simulink library "xrbsComm_r4"  (Simulink 7.1)
PreLoadFcn:
  | warning('off','MATLAB:mex:deprecatedExtension');xlmeta;com.xilinx.sysgen.util.StrategyUtil.loadAllStrategyNames();
undefined symbols (not defined in the file or in its folder): calc_path_data, gcbh, mfcm_matrix_rom, oct2dec, xlBlockLoadCallback
libraries: xbsIndex_r4 x851, mfcm_block_lib_v1 x5, xrbsComm_r4 x1, mfcm_misc_lib_v1 x1
(part 2 of 8)

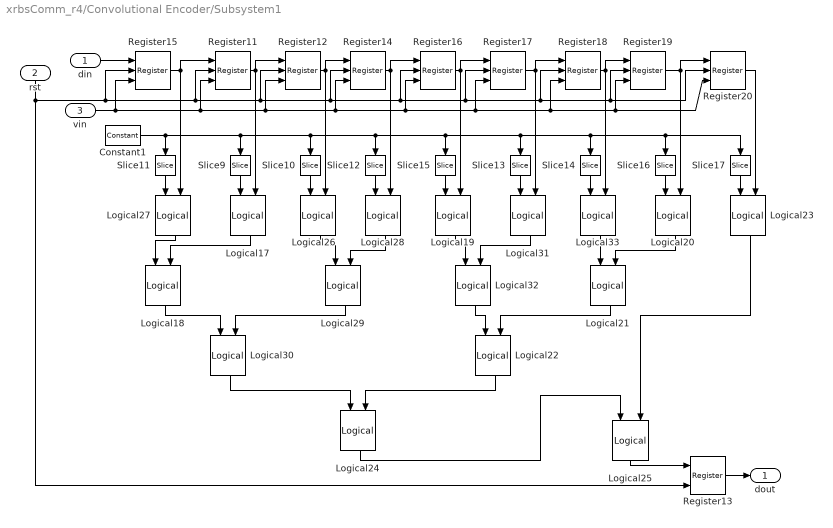
== system xrbsComm_r4/Convolutional Encoder/Subsystem1 ==
  din : Inport  OutDataType=sfix(16)  OutScaling=2^0
  rst : Inport  Orientation=down  Port=2  OutDataType=sfix(16)  OutScaling=2^0
  vin : Inport  Port=3  OutDataType=sfix(16)  OutScaling=2^0
  Constant1 : xbsIndex_r4/Constant  arith_type=Unsigned  const=oct2dec(code(index))*2^(9-K)  n_bits=9  bin_pt=0  explicit_period=off  period=1  equ=P=C  opselect=C  inp2=PCIN>>17  opr=+  inp1=P  carry=CIN  dbl_ovrd=off  block_type=constant
      settings: block_version=VER_STRING_GOES_HERE
  Logical{17,19..20,23,26..28,31,33} (9 alike) : xbsIndex_r4/Logical  Orientation=down  logical_function=AND  inputs=2  en=off  latency=0  precision=Full  arith_type=Unsigned  n_bits=16  bin_pt=0  align_bp=on  dbl_ovrd=off  block_type=logical
      settings: block_version=VER_STRING_GOES_HERE
  Logical{18,21..22,24..25,29..30,32} (8 alike) : xbsIndex_r4/Logical  Orientation=down  logical_function=XOR  inputs=2  en=off  latency=0  precision=Full  arith_type=Unsigned  n_bits=16  bin_pt=0  align_bp=on  dbl_ovrd=off  block_type=logical
      settings: block_version=VER_STRING_GOES_HERE
  Register{11..12,14..20} (9 alike) : xbsIndex_r4/Register  init=0  rst=on  en=on  dbl_ovrd=off  block_type=register
      settings: block_version=VER_STRING_GOES_HERE
  Register13 : xbsIndex_r4/Register  init=0  rst=on  en=off  dbl_ovrd=off  block_type=register
      settings: block_version=VER_STRING_GOES_HERE
  Slice10 : xbsIndex_r4/Slice  Orientation=down  nbits=1  boolean_output=off  mode=Upper Bit Location + Width  bit1=6  base1=LSB of Input  bit0=0  base0=LSB of Input  dbl_ovrd=off  block_type=slice
      settings: infoedit="Extracts a given range of bits from each input sample and presents it at the output.  The output type is ordinarily unsigned with binary point at zero, but can be Boolean when the slice is one bit wide.<P><P>Hardware notes: In hardware this block costs nothing."  block_version=VER_STRING_GOES_HERE
  Slice11 : xbsIndex_r4/Slice  Orientation=down  nbits=1  boolean_output=off  mode=Upper Bit Location + Width  bit1=8  base1=LSB of Input  bit0=0  base0=LSB of Input  dbl_ovrd=off  block_type=slice
      settings: infoedit="Extracts a given range of bits from each input sample and presents it at the output.  The output type is ordinarily unsigned with binary point at zero, but can be Boolean when the slice is one bit wide.<P><P>Hardware notes: In hardware this block costs nothing."  block_version=VER_STRING_GOES_HERE
  Slice12 : xbsIndex_r4/Slice  Orientation=down  nbits=1  boolean_output=off  mode=Upper Bit Location + Width  bit1=5  base1=LSB of Input  bit0=0  base0=LSB of Input  dbl_ovrd=off  block_type=slice
      settings: infoedit="Extracts a given range of bits from each input sample and presents it at the output.  The output type is ordinarily unsigned with binary point at zero, but can be Boolean when the slice is one bit wide.<P><P>Hardware notes: In hardware this block costs nothing."  block_version=VER_STRING_GOES_HERE
  Slice13 : xbsIndex_r4/Slice  Orientation=down  nbits=1  boolean_output=off  mode=Upper Bit Location + Width  bit1=3  base1=LSB of Input  bit0=0  base0=LSB of Input  dbl_ovrd=off  block_type=slice
      settings: infoedit="Extracts a given range of bits from each input sample and presents it at the output.  The output type is ordinarily unsigned with binary point at zero, but can be Boolean when the slice is one bit wide.<P><P>Hardware notes: In hardware this block costs nothing."  block_version=VER_STRING_GOES_HERE
  Slice14 : xbsIndex_r4/Slice  Orientation=down  nbits=1  boolean_output=off  mode=Upper Bit Location + Width  bit1=2  base1=LSB of Input  bit0=0  base0=LSB of Input  dbl_ovrd=off  block_type=slice
      settings: infoedit="Extracts a given range of bits from each input sample and presents it at the output.  The output type is ordinarily unsigned with binary point at zero, but can be Boolean when the slice is one bit wide.<P><P>Hardware notes: In hardware this block costs nothing."  block_version=VER_STRING_GOES_HERE
  Slice15 : xbsIndex_r4/Slice  Orientation=down  nbits=1  boolean_output=off  mode=Upper Bit Location + Width  bit1=4  base1=LSB of Input  bit0=0  base0=LSB of Input  dbl_ovrd=off  block_type=slice
      settings: infoedit="Extracts a given range of bits from each input sample and presents it at the output.  The output type is ordinarily unsigned with binary point at zero, but can be Boolean when the slice is one bit wide.<P><P>Hardware notes: In hardware this block costs nothing."  block_version=VER_STRING_GOES_HERE
  Slice16 : xbsIndex_r4/Slice  Orientation=down  nbits=1  boolean_output=off  mode=Upper Bit Location + Width  bit1=1  base1=LSB of Input  bit0=0  base0=LSB of Input  dbl_ovrd=off  block_type=slice
      settings: infoedit="Extracts a given range of bits from each input sample and presents it at the output.  The output type is ordinarily unsigned with binary point at zero, but can be Boolean when the slice is one bit wide.<P><P>Hardware notes: In hardware this block costs nothing."  block_version=VER_STRING_GOES_HERE
  Slice17 : xbsIndex_r4/Slice  Orientation=down  nbits=1  boolean_output=off  mode=Upper Bit Location + Width  bit1=0  base1=LSB of Input  bit0=0  base0=LSB of Input  dbl_ovrd=off  block_type=slice
      settings: infoedit="Extracts a given range of bits from each input sample and presents it at the output.  The output type is ordinarily unsigned with binary point at zero, but can be Boolean when the slice is one bit wide.<P><P>Hardware notes: In hardware this block costs nothing."  block_version=VER_STRING_GOES_HERE
  Slice9 : xbsIndex_r4/Slice  Orientation=down  nbits=1  boolean_output=off  mode=Upper Bit Location + Width  bit1=7  base1=LSB of Input  bit0=0  base0=LSB of Input  dbl_ovrd=off  block_type=slice
      settings: infoedit="Extracts a given range of bits from each input sample and presents it at the output.  The output type is ordinarily unsigned with binary point at zero, but can be Boolean when the slice is one bit wide.<P><P>Hardware notes: In hardware this block costs nothing."  block_version=VER_STRING_GOES_HERE
  dout : Outport  OutDataType=sfix(16)  OutScaling=2^0
  wires:
  Register12/1 -> Logical26/2, Register14/1
  Slice9/1 -> Logical17/1
  Slice10/1 -> Logical26/1
  Constant1/1 -> Slice9/1, Slice10/1, Slice12/1, Slice13/1, Slice14/1, Slice16/1, Slice17/1, Slice15/1, Slice11/1
  Slice11/1 -> Logical27/1
  Logical27/1 -> Logical18/1
  Logical17/1 -> Logical18/2
  Slice12/1 -> Logical28/1
  Logical26/1 -> Logical29/1
  Logical28/1 -> Logical29/2
  Logical18/1 -> Logical30/1
  Logical29/1 -> Logical30/2
  Register17/1 -> Logical31/2, Register18/1
  Register19/1 -> Logical20/2, Register20/1
  Register18/1 -> Register19/1, Logical33/2
  Slice13/1 -> Logical31/1
  Slice14/1 -> Logical33/1
  Slice15/1 -> Logical19/1
  Logical19/1 -> Logical32/1
  Logical31/1 -> Logical32/2
  Slice16/1 -> Logical20/1
  Logical33/1 -> Logical21/1
  Logical20/1 -> Logical21/2
  Logical32/1 -> Logical22/1
  Logical21/1 -> Logical22/2
  Register16/1 -> Logical19/2, Register17/1
  Register20/1 -> Logical23/2
  Slice17/1 -> Logical23/1
  Logical30/1 -> Logical24/1
  Logical22/1 -> Logical24/2
  Logical23/1 -> Logical25/2
  Logical24/1 -> Logical25/1
  Register15/1 -> Register11/1, Logical27/2
  Register14/1 -> Logical28/2, Register16/1
  Register11/1 -> Logical17/2, Register12/1
  Logical25/1 -> Register13/1
  din/1 -> Register15/1
  rst/1 -> Register11/2, Register16/2, Register18/2, Register20/2, Register19/2, Register17/2, Register14/2, Register12/2, Register15/2, Register13/2
  vin/1 -> Register20/3, Register19/3, Register18/3, Register17/3, Register16/3, Register14/3, Register12/3, Register11/3, Register15/3
  Register13/1 -> dout/1

== system xrbsComm_r4/Convolutional Encoder/Valid Out Logic ==
  vin : Inport  OutDataType=sfix(16)  OutScaling=2^0
  rst : Inport  Port=2  OutDataType=sfix(16)  OutScaling=2^0
  Register8 : xbsIndex_r4/Register  init=0  rst=on  en=off  dbl_ovrd=off  block_type=register
      settings: block_version=VER_STRING_GOES_HERE
  Register9 : xbsIndex_r4/Register  init=0  rst=on  en=off  dbl_ovrd=off  block_type=register
      settings: block_version=VER_STRING_GOES_HERE
  vout : Outport  OutDataType=sfix(16)  OutScaling=2^0
  wires:
  Register9/1 -> vout/1
  rst/1 -> Register9/2, Register8/2
  vin/1 -> Register8/1
  Register8/1 -> Register9/1

== system xrbsComm_r4/Multipath Fading Channel Model/matrix ops ==
  in_fd : Inport  OutDataType=sfix(16)  OutScaling=2^0
  in_rd : Inport  Port=2  OutDataType=sfix(16)  OutScaling=2^0
  in_reim : Inport  Port=3  OutDataType=sfix(16)  OutScaling=2^0
  fading_matrix : mfcm_block_lib_v1/fading_matrix  RATE=RATE  DATAPATH_WIDTH=DATAPATH_WIDTH  OUT_BINPT=FADE_BINPT  SPEC_DATA=SPEC_DATA  SEED=SEED
  matrix ROM : mfcm_block_lib_v1/matrix ROM  MATS=MATS  DATAPATH_WIDTH=DATAPATH_WIDTH  MAT_BINPT=MAT_BINPT
  rx_matrix : mfcm_block_lib_v1/rx_matrix  MR=size(RR,1)  N=length(GAIN)  BYPASS=MATS.rr_unity  WIDTH=DATAPATH_WIDTH  BINPT=RX_BINPT
  tx_matrix : mfcm_block_lib_v1/tx_matrix  MT=size(RT,1)  N=length(GAIN)  BYPASS=MATS.rt_unity  WIDTH=DATAPATH_WIDTH  BINPT=TX_BINPT
  out_fd : Outport  OutDataType=sfix(16)  OutScaling=2^0
  out_rd : Outport  Port=2  OutDataType=sfix(16)  OutScaling=2^0
  out_reim : Outport  Port=3  OutDataType=sfix(16)  OutScaling=2^0
  wires:
  tx_matrix/1 -> fading_matrix/1
  tx_matrix/2 -> fading_matrix/2
  tx_matrix/3 -> fading_matrix/3
  fading_matrix/1 -> rx_matrix/1
  fading_matrix/2 -> rx_matrix/2
  fading_matrix/3 -> rx_matrix/3
  rx_matrix/4 -> matrix ROM/1
  tx_matrix/4 -> matrix ROM/2
  matrix ROM/1 -> rx_matrix/4
  matrix ROM/2 -> tx_matrix/4
  rx_matrix/1 -> out_fd/1
  in_fd/1 -> tx_matrix/1
  rx_matrix/2 -> out_rd/1
  in_rd/1 -> tx_matrix/2
  rx_matrix/3 -> out_reim/1
  in_reim/1 -> tx_matrix/3

== system xrbsComm_r4/White Gaussian  Noise Generator/Box-Muller1 ==
  " reset" : Inport  OutDataType=sfix(16)  OutScaling=2^0
  Convert : xbsIndex_r4/Convert  arith_type="Signed  (2's comp)"  n_bits=10  bin_pt=6  quantization="Round  (unbiased: +/- Inf)"  overflow=Wrap  latency=2  dbl_ovrd=off  pipeline=off  block_type=convert
      settings: infoedit=The input is presented at the output after quantization and overflow effects.<P><P>Hardware notes: Additional hardware is used when rounding or saturation is selected and output width is less than the input width.  xl_area=[0, 0, 0, 0, 0, 0, 0]  block_version=VER_STRING_GOES_HERE
  Mult : xbsIndex_r4/Mult  precision=Full  arith_type="Signed  (2's comp)"  n_bits=20  bin_pt=0  quantization="Round  (unbiased: +/- Inf)"  overflow=Wrap  en=off  latency=2  dbl_ovrd=off  use_behavioral_HDL=off  use_embedded=on  pipeline=on  use_rpm=off  placement_style=Rectangular shape  block_type=mult
      settings: infoedit=Multiplies two values.<P><P>Hardware notes: To use the internal pipeline stage of the dedicated multiplier you must select 'Pipeline to Greatest Extent Possible'.  xl_area=[0, 0, 0, 0, 0, 0, 0]  block_version=VER_STRING_GOES_HERE
  f : Subsystem  mask(f_rom){init1=f_init1, init2=f_init2, init3=f_init3, init4=f_init4, init5=f_init5}
      mask prompts: init1 "init1(17:1)"; init2 "init2(25:1)"; init3 "init3(29:1)"; init4 "init4(31:1)"; init5 "init5(41:1)"
  g : Subsystem  mask{init=g_init}
      mask prompts: init "g_init(47:1)"
  bm : Outport  OutDataType=sfix(16)  OutScaling=2^0
  wires:
  g/1(g(s')) -> Mult/2
  f/1(f(s')) -> Mult/1
  Mult/1 -> Convert/1
  Convert/1 -> bm/1
  " reset"/1 -> f/1("reset "), g/1(reset)

== system xrbsComm_r4/White Gaussian  Noise Generator/Box-Muller2 ==
  reset : Inport  OutDataType=sfix(16)  OutScaling=2^0
  Convert : xbsIndex_r4/Convert  arith_type="Signed  (2's comp)"  n_bits=10  bin_pt=6  quantization="Round  (unbiased: +/- Inf)"  overflow=Wrap  latency=2  dbl_ovrd=off  pipeline=off  block_type=convert
      settings: infoedit=The input is presented at the output after quantization and overflow effects.<P><P>Hardware notes: Additional hardware is used when rounding or saturation is selected and output width is less than the input width.  xl_area=[0, 0, 0, 0, 0, 0, 0]  block_version=VER_STRING_GOES_HERE
  Mult : xbsIndex_r4/Mult  precision=Full  arith_type="Signed  (2's comp)"  n_bits=20  bin_pt=0  quantization="Round  (unbiased: +/- Inf)"  overflow=Wrap  en=off  latency=2  dbl_ovrd=off  use_behavioral_HDL=off  use_embedded=on  pipeline=on  use_rpm=off  placement_style=Rectangular shape  block_type=mult
      settings: infoedit=Multiplies two values.<P><P>Hardware notes: To use the internal pipeline stage of the dedicated multiplier you must select 'Pipeline to Greatest Extent Possible'.  xl_area=[0, 0, 0, 0, 0, 0, 0]  block_version=VER_STRING_GOES_HERE
  fr1 : Subsystem  mask(f_rom){init1=f_init1, init2=f_init2, init3=f_init3, init4=f_init4, init5=f_init5}
      mask prompts: init1 "init1(17:1)"; init2 "init2(25:1)"; init3 "init3(29:1)"; init4 "init4(31:1)"; init5 "init5(41:1)"
  g2 : Subsystem  mask{init=g_init}
      mask prompts: init "g_init(47:1)"
  bm : Outport  OutDataType=sfix(16)  OutScaling=2^0
  wires:
  g2/1(g(s')) -> Mult/2
  Mult/1 -> Convert/1
  Convert/1 -> bm/1
  reset/1 -> fr1/1(reset), g2/1(reset)
  fr1/1(f(s')) -> Mult/1

== system xrbsComm_r4/White Gaussian  Noise Generator/Box-Muller3 ==
  reset : Inport  OutDataType=sfix(16)  OutScaling=2^0
  Convert : xbsIndex_r4/Convert  arith_type="Signed  (2's comp)"  n_bits=10  bin_pt=6  quantization="Round  (unbiased: +/- Inf)"  overflow=Wrap  latency=2  dbl_ovrd=off  pipeline=off  block_type=convert
      settings: infoedit=The input is presented at the output after quantization and overflow effects.<P><P>Hardware notes: Additional hardware is used when rounding or saturation is selected and output width is less than the input width.  xl_area=[0, 0, 0, 0, 0, 0, 0]  block_version=VER_STRING_GOES_HERE
  Mult : xbsIndex_r4/Mult  precision=Full  arith_type="Signed  (2's comp)"  n_bits=20  bin_pt=0  quantization="Round  (unbiased: +/- Inf)"  overflow=Wrap  en=off  latency=2  dbl_ovrd=off  use_behavioral_HDL=off  use_embedded=on  pipeline=on  use_rpm=off  placement_style=Rectangular shape  block_type=mult
      settings: infoedit=Multiplies two values.<P><P>Hardware notes: To use the internal pipeline stage of the dedicated multiplier you must select 'Pipeline to Greatest Extent Possible'.  xl_area=[0, 0, 0, 0, 0, 0, 0]  block_version=VER_STRING_GOES_HERE
  fr1 : Subsystem  mask(f_rom){init1=f_init1, init2=f_init2, init3=f_init3, init4=f_init4, init5=f_init5}
      mask prompts: init1 "init1(17:1)"; init2 "init2(25:1)"; init3 "init3(29:1)"; init4 "init4(31:1)"; init5 "init5(41:1)"
  g2 : Subsystem  mask{init=g_init}
      mask prompts: init "g_init(47:1)"
  bm : Outport  OutDataType=sfix(16)  OutScaling=2^0
  wires:
  g2/1(g(s')) -> Mult/2
  fr1/1(f(s')) -> Mult/1
  Mult/1 -> Convert/1
  Convert/1 -> bm/1
  reset/1 -> fr1/1(reset), g2/1(reset)

== system xrbsComm_r4/White Gaussian  Noise Generator/Box-Muller4 ==
  reset : Inport  OutDataType=sfix(16)  OutScaling=2^0
  Convert : xbsIndex_r4/Convert  arith_type="Signed  (2's comp)"  n_bits=10  bin_pt=6  quantization="Round  (unbiased: +/- Inf)"  overflow=Wrap  latency=2  dbl_ovrd=off  pipeline=off  block_type=convert
      settings: infoedit=The input is presented at the output after quantization and overflow effects.<P><P>Hardware notes: Additional hardware is used when rounding or saturation is selected and output width is less than the input width.  xl_area=[0, 0, 0, 0, 0, 0, 0]  block_version=VER_STRING_GOES_HERE
  Mult : xbsIndex_r4/Mult  precision=Full  arith_type="Signed  (2's comp)"  n_bits=20  bin_pt=0  quantization="Round  (unbiased: +/- Inf)"  overflow=Wrap  en=off  latency=2  dbl_ovrd=off  use_behavioral_HDL=off  use_embedded=on  pipeline=on  use_rpm=off  placement_style=Rectangular shape  block_type=mult
      settings: infoedit=Multiplies two values.<P><P>Hardware notes: To use the internal pipeline stage of the dedicated multiplier you must select 'Pipeline to Greatest Extent Possible'.  xl_area=[0, 0, 0, 0, 0, 0, 0]  block_version=VER_STRING_GOES_HERE
  fr1 : Subsystem  mask(f_rom){init1=f_init1, init2=f_init2, init3=f_init3, init4=f_init4, init5=f_init5}
      mask prompts: init1 "init1(17:1)"; init2 "init2(25:1)"; init3 "init3(29:1)"; init4 "init4(31:1)"; init5 "init5(41:1)"
  g2 : Subsystem  mask{init=g_init}
      mask prompts: init "g_init(47:1)"
  bm : Outport  OutDataType=sfix(16)  OutScaling=2^0
  wires:
  reset/1 -> g2/1(reset), fr1/1(reset)
  g2/1(g(s')) -> Mult/2
  fr1/1(f(s')) -> Mult/1
  Mult/1 -> Convert/1
  Convert/1 -> bm/1

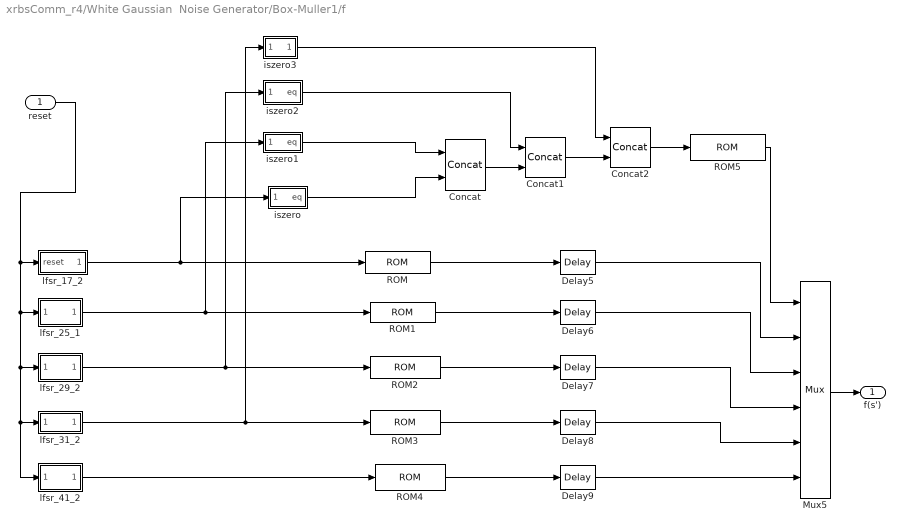
== system xrbsComm_r4/White Gaussian  Noise Generator/Box-Muller1/f ==
  "reset " : Inport  OutDataType=sfix(16)  OutScaling=2^0
  Concat : xbsIndex_r4/Concat  num_inputs=2  dbl_ovrd=off  block_type=concat
      settings: block_version=VER_STRING_GOES_HERE
  Concat1 : xbsIndex_r4/Concat  num_inputs=2  dbl_ovrd=off  block_type=concat
      settings: block_version=VER_STRING_GOES_HERE
  Concat2 : xbsIndex_r4/Concat  num_inputs=2  dbl_ovrd=off  block_type=concat
      settings: block_version=VER_STRING_GOES_HERE
  Delay{5..9} (5 alike) : xbsIndex_r4/Delay  en=off  latency=2  dbl_ovrd=off  reg_retiming=off  block_type=delay
      settings: infoedit="Delay line having  configurable length.<P><P>Hardware notes: A delay line is a chain, each link of which is an SRL16 followed by a flip-flop. If register retiming is enabled, the delay line is a chain of flip-flops."  xl_area=[0, 0, 0, 0, 0, 0, 0]  block_version=VER_STRING_GOES_HERE
  Mux5 : xbsIndex_r4/Mux  inputs=5  en=off  latency=1  precision=Full  arith_type="Signed  (2's comp)"  n_bits=10  bin_pt=0  quantization="Round  (unbiased: +/- Inf)"  overflow=Wrap  dbl_ovrd=off  block_type=mux
      settings: xl_area=[0, 0, 0, 0, 0, 0, 0]  block_version=VER_STRING_GOES_HERE
  ROM : xbsIndex_r4/ROM  depth=16  initVector=sqrt(-log( ((0:15)+0.51)'*(2.^(-1.*4)) ))  distributed_mem=Distributed memory  rst=off  init_reg=0  en=off  latency=1  arith_type=Unsigned  n_bits=9  bin_pt=7  dbl_ovrd=off  use_rpm=off  block_type=sprom
      settings: xl_area=[0, 0, 0, 0, 0, 0, 0]  block_version=VER_STRING_GOES_HERE
  ROM1 : xbsIndex_r4/ROM  depth=16  initVector=sqrt(-log( ((0:15)+0.51)'*(2.^(-2.*4)) ))  distributed_mem=Distributed memory  rst=off  init_reg=0  en=off  latency=1  arith_type=Unsigned  n_bits=9  bin_pt=7  dbl_ovrd=off  use_rpm=off  block_type=sprom
      settings: xl_area=[0, 0, 0, 0, 0, 0, 0]  block_version=VER_STRING_GOES_HERE
  ROM2 : xbsIndex_r4/ROM  depth=16  initVector=sqrt(-log( ((0:15)+0.51)'*(2.^(-3.*4)) ))  distributed_mem=Distributed memory  rst=off  init_reg=0  en=off  latency=1  arith_type=Unsigned  n_bits=9  bin_pt=7  dbl_ovrd=off  use_rpm=off  block_type=sprom
      settings: xl_area=[0, 0, 0, 0, 0, 0, 0]  block_version=VER_STRING_GOES_HERE
  ROM3 : xbsIndex_r4/ROM  depth=16  initVector=sqrt(-log( ((0:15)+0.51)'*(2.^(-4.*4)) ))  distributed_mem=Distributed memory  rst=off  init_reg=0  en=off  latency=1  arith_type=Unsigned  n_bits=9  bin_pt=7  dbl_ovrd=off  use_rpm=off  block_type=sprom
      settings: xl_area=[0, 0, 0, 0, 0, 0, 0]  block_version=VER_STRING_GOES_HERE
  ROM4 : xbsIndex_r4/ROM  depth=16  initVector=sqrt(-log( ((0:15)+0.51)'*(2.^(-5.*4)) ))  distributed_mem=Distributed memory  rst=off  init_reg=0  en=off  latency=1  arith_type=Unsigned  n_bits=9  bin_pt=7  dbl_ovrd=off  use_rpm=off  block_type=sprom
      settings: xl_area=[0, 0, 0, 0, 0, 0, 0]  block_version=VER_STRING_GOES_HERE
  ROM5 : xbsIndex_r4/ROM  depth=16  initVector=[0 1 0 2 0 1 0 3 0 1 0 2 0 1 0 4]  distributed_mem=Block RAM  rst=off  init_reg=0  en=off  latency=2  arith_type=Unsigned  n_bits=3  bin_pt=0  dbl_ovrd=off  use_rpm=off  block_type=sprom
      settings: xl_area=[0, 0, 0, 0, 0, 0, 0]  block_version=VER_STRING_GOES_HERE
  iszero : Subsystem
  iszero1 : Subsystem
  iszero2 : Subsystem
  iszero3 : Subsystem
  lfsr_17_2 : Subsystem  mask(lfsr_17){init=init1}
      mask prompts: init "init(17:1)"
  lfsr_25_1 : Subsystem  mask(lfsr_25){init=init2}
      mask prompts: init "init(25:1)"
  lfsr_29_2 : Subsystem  mask(lfsr_29){init=init3}
      mask prompts: init "init(29:1)"
  lfsr_31_2 : Subsystem  mask(lfsr_31){init=init4}
      mask prompts: init "init(31:1)"
  lfsr_41_2 : Subsystem  mask(lfsr_41){init=init5}
      mask prompts: init "init(41:1)"
  f(s') : Outport  OutDataType=sfix(16)  OutScaling=2^0
  wires:
  lfsr_17_2/1(" ") -> ROM/1, iszero/1(" ")
  lfsr_25_1/1(" ") -> ROM1/1, iszero1/1(" ")
  lfsr_29_2/1(" ") -> ROM2/1, iszero2/1(" ")
  lfsr_31_2/1(" ") -> iszero3/1(" "), ROM3/1
  lfsr_41_2/1(" ") -> ROM4/1
  Concat2/1 -> ROM5/1
  ROM5/1 -> Mux5/1
  Concat/1 -> Concat1/2
  Concat1/1 -> Concat2/2
  Mux5/1 -> f(s')/1
  ROM/1 -> Delay5/1
  ROM1/1 -> Delay6/1
  ROM2/1 -> Delay7/1
  ROM3/1 -> Delay8/1
  ROM4/1 -> Delay9/1
  iszero/1(eq) -> Concat/2
  iszero1/1(eq) -> Concat/1
  iszero2/1(eq) -> Concat1/1
  iszero3/1(eq) -> Concat2/1
  Delay5/1 -> Mux5/2
  Delay6/1 -> Mux5/3
  Delay7/1 -> Mux5/4
  Delay8/1 -> Mux5/5
  Delay9/1 -> Mux5/6
  "reset "/1 -> lfsr_25_1/1(" reset"), lfsr_41_2/1(reset), lfsr_31_2/1(reset), lfsr_29_2/1(reset), lfsr_17_2/1(reset)

== system xrbsComm_r4/White Gaussian  Noise Generator/Box-Muller1/g ==
  reset : Inport  OutDataType=sfix(16)  OutScaling=2^0
  Delay : xbsIndex_r4/Delay  en=off  latency=3  dbl_ovrd=off  reg_retiming=off  block_type=delay
      settings: infoedit="Delay line having  configurable length.<P><P>Hardware notes: A delay line is a chain, each link of which is an SRL16 followed by a flip-flop. If register retiming is enabled, the delay line is a chain of flip-flops."  xl_area=[0, 0, 0, 0, 0, 0, 0]  block_version=VER_STRING_GOES_HERE
  ROM : xbsIndex_r4/ROM  depth=256  initVector=sqrt(2) * cos(pi*((0:255) + 0.5)*2^(-8))  distributed_mem=Block RAM  rst=off  init_reg=0  en=off  latency=1  arith_type="Signed  (2's comp)"  n_bits=10  bin_pt=8  dbl_ovrd=off  use_rpm=off  block_type=sprom
      settings: xl_area=[0, 0, 0, 0, 0, 0, 0]  block_version=VER_STRING_GOES_HERE
  lfsr_47_5 : Subsystem  mask(lfsr_47){init=init}
      mask prompts: init "init(47:1)"
  g(s') : Outport  OutDataType=sfix(16)  OutScaling=2^0
  wires:
  ROM/1 -> Delay/1
  lfsr_47_5/1(" ") -> ROM/1
  Delay/1 -> g(s')/1
  reset/1 -> lfsr_47_5/1(reset)

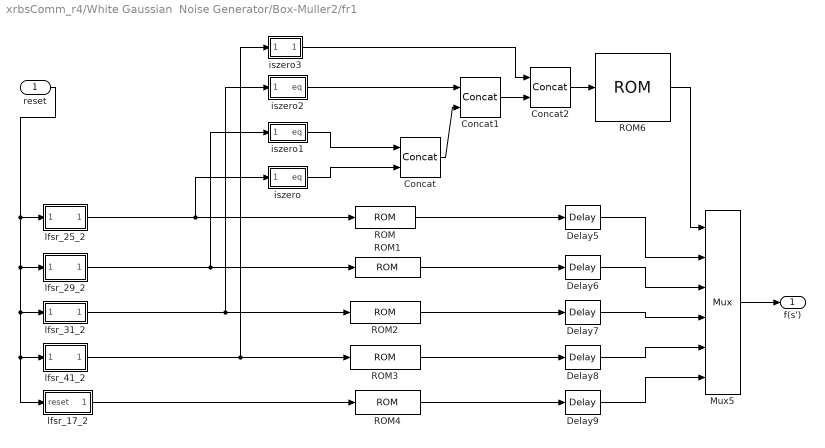
== system xrbsComm_r4/White Gaussian  Noise Generator/Box-Muller2/fr1 ==
  reset : Inport  OutDataType=sfix(16)  OutScaling=2^0
  Concat : xbsIndex_r4/Concat  num_inputs=2  dbl_ovrd=off  block_type=concat
      settings: block_version=VER_STRING_GOES_HERE
  Concat1 : xbsIndex_r4/Concat  num_inputs=2  dbl_ovrd=off  block_type=concat
      settings: block_version=VER_STRING_GOES_HERE
  Concat2 : xbsIndex_r4/Concat  num_inputs=2  dbl_ovrd=off  block_type=concat
      settings: block_version=VER_STRING_GOES_HERE
  Delay{5..9} (5 alike) : xbsIndex_r4/Delay  en=off  latency=2  dbl_ovrd=off  reg_retiming=off  block_type=delay
      settings: infoedit="Delay line having  configurable length.<P><P>Hardware notes: A delay line is a chain, each link of which is an SRL16 followed by a flip-flop. If register retiming is enabled, the delay line is a chain of flip-flops."  xl_area=[0, 0, 0, 0, 0, 0, 0]  block_version=VER_STRING_GOES_HERE
  Mux5 : xbsIndex_r4/Mux  inputs=5  en=off  latency=1  precision=Full  arith_type="Signed  (2's comp)"  n_bits=10  bin_pt=0  quantization="Round  (unbiased: +/- Inf)"  overflow=Wrap  dbl_ovrd=off  block_type=mux
      settings: xl_area=[0, 0, 0, 0, 0, 0, 0]  block_version=VER_STRING_GOES_HERE
  ROM : xbsIndex_r4/ROM  depth=16  initVector=sqrt(-log( ((0:15)+0.51)'*(2.^(-1.*4)) ))  distributed_mem=Distributed memory  rst=off  init_reg=0  en=off  latency=1  arith_type=Unsigned  n_bits=9  bin_pt=7  dbl_ovrd=off  use_rpm=off  block_type=sprom
      settings: xl_area=[0, 0, 0, 0, 0, 0, 0]  block_version=VER_STRING_GOES_HERE
  ROM1 : xbsIndex_r4/ROM  depth=16  initVector=sqrt(-log( ((0:15)+0.51)'*(2.^(-2.*4)) ))  distributed_mem=Distributed memory  rst=off  init_reg=0  en=off  latency=1  arith_type=Unsigned  n_bits=9  bin_pt=7  dbl_ovrd=off  use_rpm=off  block_type=sprom
      settings: xl_area=[0, 0, 0, 0, 0, 0, 0]  block_version=VER_STRING_GOES_HERE
  ROM2 : xbsIndex_r4/ROM  depth=16  initVector=sqrt(-log( ((0:15)+0.51)'*(2.^(-3.*4)) ))  distributed_mem=Distributed memory  rst=off  init_reg=0  en=off  latency=1  arith_type=Unsigned  n_bits=9  bin_pt=7  dbl_ovrd=off  use_rpm=off  block_type=sprom
      settings: xl_area=[0, 0, 0, 0, 0, 0, 0]  block_version=VER_STRING_GOES_HERE
  ROM3 : xbsIndex_r4/ROM  depth=16  initVector=sqrt(-log( ((0:15)+0.51)'*(2.^(-4.*4)) ))  distributed_mem=Distributed memory  rst=off  init_reg=0  en=off  latency=1  arith_type=Unsigned  n_bits=9  bin_pt=7  dbl_ovrd=off  use_rpm=off  block_type=sprom
      settings: xl_area=[0, 0, 0, 0, 0, 0, 0]  block_version=VER_STRING_GOES_HERE
  ROM4 : xbsIndex_r4/ROM  depth=16  initVector=sqrt(-log( ((0:15)+0.51)'*(2.^(-5.*4)) ))  distributed_mem=Distributed memory  rst=off  init_reg=0  en=off  latency=1  arith_type=Unsigned  n_bits=9  bin_pt=7  dbl_ovrd=off  use_rpm=off  block_type=sprom
      settings: xl_area=[0, 0, 0, 0, 0, 0, 0]  block_version=VER_STRING_GOES_HERE
  ROM6 : xbsIndex_r4/ROM  depth=16  initVector=[0 1 0 2 0 1 0 3 0 1 0 2 0 1 0 4]  distributed_mem=Block RAM  rst=off  init_reg=0  en=off  latency=2  arith_type=Unsigned  n_bits=3  bin_pt=0  dbl_ovrd=off  use_rpm=off  block_type=sprom
      settings: xl_area=[0, 0, 0, 0, 0, 0, 0]  block_version=VER_STRING_GOES_HERE
  iszero : Subsystem
  iszero1 : Subsystem
  iszero2 : Subsystem
  iszero3 : Subsystem
  lfsr_17_2 : Subsystem  mask(lfsr_17){init=init1}
      mask prompts: init "init(17:1)"
  lfsr_25_2 : Subsystem  mask(lfsr_25){init=init2}
      mask prompts: init "init(25:1)"
  lfsr_29_2 : Subsystem  mask(lfsr_29){init=init3}
      mask prompts: init "init(29:1)"
  lfsr_31_2 : Subsystem  mask(lfsr_31){init=init4}
      mask prompts: init "init(31:1)"
  lfsr_41_2 : Subsystem  mask(lfsr_41){init=init5}
      mask prompts: init "init(41:1)"
  f(s') : Outport  OutDataType=sfix(16)  OutScaling=2^0
  wires:
  Delay9/1 -> Mux5/6
  Delay8/1 -> Mux5/5
  Delay7/1 -> Mux5/4
  Delay6/1 -> Mux5/3
  Delay5/1 -> Mux5/2
  iszero/1(eq) -> Concat/2
  lfsr_25_2/1(" ") -> iszero/1(" "), ROM/1
  lfsr_29_2/1(" ") -> ROM1/1, iszero1/1(" ")
  lfsr_31_2/1(" ") -> iszero2/1(" "), ROM2/1
  lfsr_41_2/1(" ") -> ROM3/1, iszero3/1(" ")
  lfsr_17_2/1(" ") -> ROM4/1
  Concat/1 -> Concat1/2
  Concat1/1 -> Concat2/2
  ROM/1 -> Delay5/1
  ROM1/1 -> Delay6/1
  ROM4/1 -> Delay9/1
  ROM6/1 -> Mux5/1
  iszero1/1(eq) -> Concat/1
  Concat2/1 -> ROM6/1
  iszero2/1(eq) -> Concat1/1
  iszero3/1(eq) -> Concat2/1
  ROM2/1 -> Delay7/1
  ROM3/1 -> Delay8/1
  Mux5/1 -> f(s')/1
  reset/1 -> lfsr_25_2/1(" reset"), lfsr_29_2/1(reset), lfsr_31_2/1(reset), lfsr_17_2/1(reset), lfsr_41_2/1(reset)

== system xrbsComm_r4/White Gaussian  Noise Generator/Box-Muller2/g2 ==
  reset : Inport  OutDataType=sfix(16)  OutScaling=2^0
  Delay : xbsIndex_r4/Delay  en=off  latency=3  dbl_ovrd=off  reg_retiming=off  block_type=delay
      settings: infoedit="Delay line having  configurable length.<P><P>Hardware notes: A delay line is a chain, each link of which is an SRL16 followed by a flip-flop. If register retiming is enabled, the delay line is a chain of flip-flops."  xl_area=[0, 0, 0, 0, 0, 0, 0]  block_version=VER_STRING_GOES_HERE
  ROM : xbsIndex_r4/ROM  depth=256  initVector=sqrt(2) * cos(pi*((0:255) + 0.5)*2^(-8))  distributed_mem=Block RAM  rst=off  init_reg=0  en=off  latency=1  arith_type="Signed  (2's comp)"  n_bits=10  bin_pt=8  dbl_ovrd=off  use_rpm=off  block_type=sprom
      settings: xl_area=[0, 0, 0, 0, 0, 0, 0]  block_version=VER_STRING_GOES_HERE
  lfsr_47_5 : Subsystem  mask(lfsr_47){init=init}
      mask prompts: init "init(47:1)"
  g(s') : Outport  OutDataType=sfix(16)  OutScaling=2^0
  wires:
  ROM/1 -> Delay/1
  lfsr_47_5/1(" ") -> ROM/1
  Delay/1 -> g(s')/1
  reset/1 -> lfsr_47_5/1(reset)

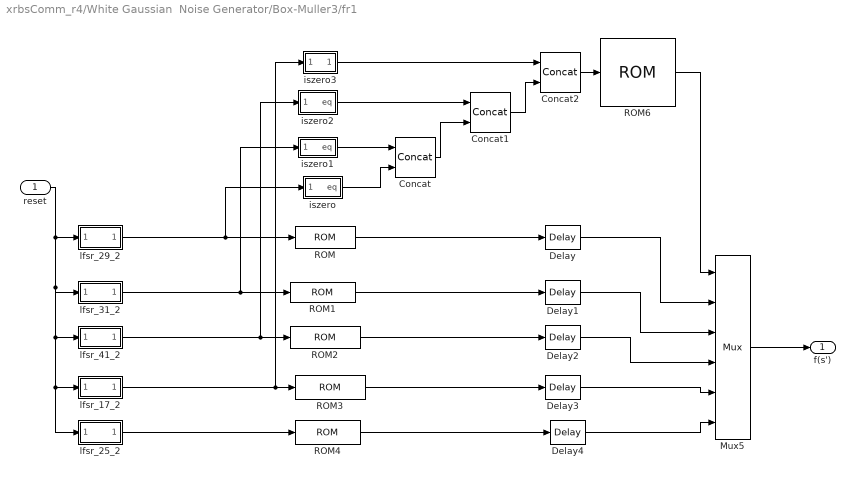
== system xrbsComm_r4/White Gaussian  Noise Generator/Box-Muller3/fr1 ==
  reset : Inport  OutDataType=sfix(16)  OutScaling=2^0
  Concat : xbsIndex_r4/Concat  num_inputs=2  dbl_ovrd=off  block_type=concat
      settings: block_version=VER_STRING_GOES_HERE
  Concat1 : xbsIndex_r4/Concat  num_inputs=2  dbl_ovrd=off  block_type=concat
      settings: block_version=VER_STRING_GOES_HERE
  Concat2 : xbsIndex_r4/Concat  num_inputs=2  dbl_ovrd=off  block_type=concat
      settings: block_version=VER_STRING_GOES_HERE
  Delay{,1..4} (5 alike) : xbsIndex_r4/Delay  en=off  latency=2  dbl_ovrd=off  reg_retiming=off  block_type=delay
      settings: infoedit="Delay line having  configurable length.<P><P>Hardware notes: A delay line is a chain, each link of which is an SRL16 followed by a flip-flop. If register retiming is enabled, the delay line is a chain of flip-flops."  xl_area=[0, 0, 0, 0, 0, 0, 0]  block_version=VER_STRING_GOES_HERE
  Mux5 : xbsIndex_r4/Mux  inputs=5  en=off  latency=1  precision=Full  arith_type="Signed  (2's comp)"  n_bits=10  bin_pt=0  quantization="Round  (unbiased: +/- Inf)"  overflow=Wrap  dbl_ovrd=off  block_type=mux
      settings: xl_area=[0, 0, 0, 0, 0, 0, 0]  block_version=VER_STRING_GOES_HERE
  ROM : xbsIndex_r4/ROM  depth=16  initVector=sqrt(-log( ((0:15)+0.51)'*(2.^(-1.*4)) ))  distributed_mem=Distributed memory  rst=off  init_reg=0  en=off  latency=1  arith_type=Unsigned  n_bits=9  bin_pt=7  dbl_ovrd=off  use_rpm=off  block_type=sprom
      settings: xl_area=[0, 0, 0, 0, 0, 0, 0]  block_version=VER_STRING_GOES_HERE
  ROM1 : xbsIndex_r4/ROM  depth=16  initVector=sqrt(-log( ((0:15)+0.51)'*(2.^(-2.*4)) ))  distributed_mem=Distributed memory  rst=off  init_reg=0  en=off  latency=1  arith_type=Unsigned  n_bits=9  bin_pt=7  dbl_ovrd=off  use_rpm=off  block_type=sprom
      settings: xl_area=[0, 0, 0, 0, 0, 0, 0]  block_version=VER_STRING_GOES_HERE
  ROM2 : xbsIndex_r4/ROM  depth=16  initVector=sqrt(-log( ((0:15)+0.51)'*(2.^(-3.*4)) ))  distributed_mem=Distributed memory  rst=off  init_reg=0  en=off  latency=1  arith_type=Unsigned  n_bits=9  bin_pt=7  dbl_ovrd=off  use_rpm=off  block_type=sprom
      settings: xl_area=[0, 0, 0, 0, 0, 0, 0]  block_version=VER_STRING_GOES_HERE
  ROM3 : xbsIndex_r4/ROM  depth=16  initVector=sqrt(-log( ((0:15)+0.51)'*(2.^(-4.*4)) ))  distributed_mem=Distributed memory  rst=off  init_reg=0  en=off  latency=1  arith_type=Unsigned  n_bits=9  bin_pt=7  dbl_ovrd=off  use_rpm=off  block_type=sprom
      settings: xl_area=[0, 0, 0, 0, 0, 0, 0]  block_version=VER_STRING_GOES_HERE
  ROM4 : xbsIndex_r4/ROM  depth=16  initVector=sqrt(-log( ((0:15)+0.51)'*(2.^(-5.*4)) ))  distributed_mem=Distributed memory  rst=off  init_reg=0  en=off  latency=1  arith_type=Unsigned  n_bits=9  bin_pt=7  dbl_ovrd=off  use_rpm=off  block_type=sprom
      settings: xl_area=[0, 0, 0, 0, 0, 0, 0]  block_version=VER_STRING_GOES_HERE
  ROM6 : xbsIndex_r4/ROM  depth=16  initVector=[0 1 0 2 0 1 0 3 0 1 0 2 0 1 0 4]  distributed_mem=Block RAM  rst=off  init_reg=0  en=off  latency=2  arith_type=Unsigned  n_bits=3  bin_pt=0  dbl_ovrd=off  use_rpm=off  block_type=sprom
      settings: xl_area=[0, 0, 0, 0, 0, 0, 0]  block_version=VER_STRING_GOES_HERE
  iszero : Subsystem
  iszero1 : Subsystem
  iszero2 : Subsystem
  iszero3 : Subsystem
  lfsr_17_2 : Subsystem  mask(lfsr_17){init=init1}
      mask prompts: init "init(17:1)"
  lfsr_25_2 : Subsystem  mask(lfsr_25){init=init2}
      mask prompts: init "init(25:1)"
  lfsr_29_2 : Subsystem  mask(lfsr_29){init=init3}
      mask prompts: init "init(29:1)"
  lfsr_31_2 : Subsystem  mask(lfsr_31){init=init4}
      mask prompts: init "init(31:1)"
  lfsr_41_2 : Subsystem  mask(lfsr_41){init=init5}
      mask prompts: init "init(41:1)"
  f(s') : Outport  OutDataType=sfix(16)  OutScaling=2^0
  wires:
  lfsr_29_2/1(" ") -> ROM/1, iszero/1(" ")
  lfsr_31_2/1(" ") -> ROM1/1, iszero1/1(" ")
  lfsr_41_2/1(" ") -> ROM2/1, iszero2/1(" ")
  lfsr_17_2/1(" ") -> iszero3/1(" "), ROM3/1
  lfsr_25_2/1(" ") -> ROM4/1
  Mux5/1 -> f(s')/1
  Concat/1 -> Concat1/2
  Concat1/1 -> Concat2/2
  Concat2/1 -> ROM6/1
  ROM6/1 -> Mux5/1
  ROM/1 -> Delay/1
  ROM1/1 -> Delay1/1
  ROM2/1 -> Delay2/1
  ROM3/1 -> Delay3/1
  ROM4/1 -> Delay4/1
  iszero/1(eq) -> Concat/2
  iszero1/1(eq) -> Concat/1
  iszero2/1(eq) -> Concat1/1
  iszero3/1(eq) -> Concat2/1
  Delay4/1 -> Mux5/6
  Delay3/1 -> Mux5/5
  Delay2/1 -> Mux5/4
  Delay1/1 -> Mux5/3
  Delay/1 -> Mux5/2
  reset/1 -> lfsr_31_2/1(reset), lfsr_41_2/1(reset), lfsr_25_2/1(" reset"), lfsr_17_2/1(reset), lfsr_29_2/1(reset)

== system xrbsComm_r4/White Gaussian  Noise Generator/Box-Muller3/g2 ==
  reset : Inport  OutDataType=sfix(16)  OutScaling=2^0
  Delay : xbsIndex_r4/Delay  en=off  latency=3  dbl_ovrd=off  reg_retiming=off  block_type=delay
      settings: infoedit="Delay line having  configurable length.<P><P>Hardware notes: A delay line is a chain, each link of which is an SRL16 followed by a flip-flop. If register retiming is enabled, the delay line is a chain of flip-flops."  xl_area=[0, 0, 0, 0, 0, 0, 0]  block_version=VER_STRING_GOES_HERE
  ROM : xbsIndex_r4/ROM  depth=256  initVector=sqrt(2) * cos(pi*((0:255) + 0.5)*2^(-8))  distributed_mem=Block RAM  rst=off  init_reg=0  en=off  latency=1  arith_type="Signed  (2's comp)"  n_bits=10  bin_pt=8  dbl_ovrd=off  use_rpm=off  block_type=sprom
      settings: xl_area=[0, 0, 0, 0, 0, 0, 0]  block_version=VER_STRING_GOES_HERE
  lfsr_47_5 : Subsystem  mask(lfsr_47){init=init}
      mask prompts: init "init(47:1)"
  g(s') : Outport  OutDataType=sfix(16)  OutScaling=2^0
  wires:
  ROM/1 -> Delay/1
  Delay/1 -> g(s')/1
  reset/1 -> lfsr_47_5/1(reset)
  lfsr_47_5/1(" ") -> ROM/1

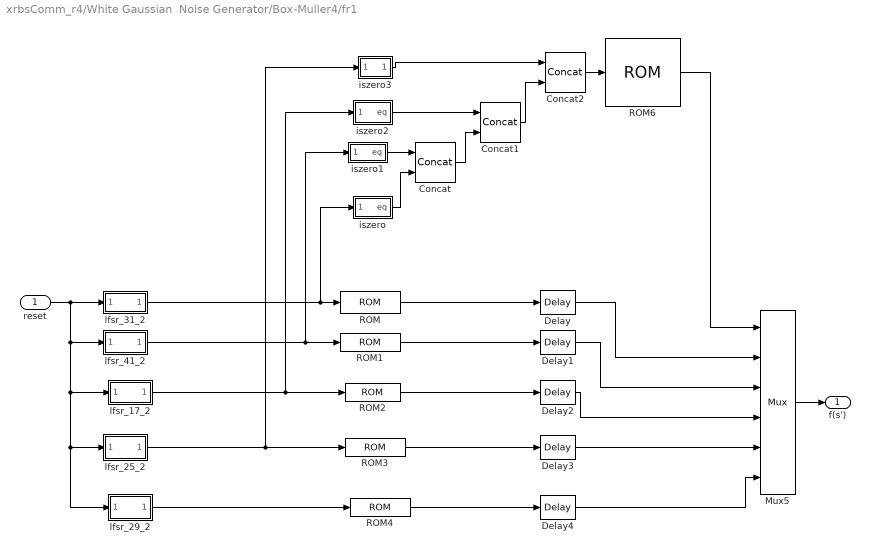
== system xrbsComm_r4/White Gaussian  Noise Generator/Box-Muller4/fr1 ==
  reset : Inport  OutDataType=sfix(16)  OutScaling=2^0
  Concat : xbsIndex_r4/Concat  num_inputs=2  dbl_ovrd=off  block_type=concat
      settings: block_version=VER_STRING_GOES_HERE
  Concat1 : xbsIndex_r4/Concat  num_inputs=2  dbl_ovrd=off  block_type=concat
      settings: block_version=VER_STRING_GOES_HERE
  Concat2 : xbsIndex_r4/Concat  num_inputs=2  dbl_ovrd=off  block_type=concat
      settings: block_version=VER_STRING_GOES_HERE
  Delay{,1..4} (5 alike) : xbsIndex_r4/Delay  en=off  latency=2  dbl_ovrd=off  reg_retiming=off  block_type=delay
      settings: infoedit="Delay line having  configurable length.<P><P>Hardware notes: A delay line is a chain, each link of which is an SRL16 followed by a flip-flop. If register retiming is enabled, the delay line is a chain of flip-flops."  xl_area=[0, 0, 0, 0, 0, 0, 0]  block_version=VER_STRING_GOES_HERE
  Mux5 : xbsIndex_r4/Mux  inputs=5  en=off  latency=1  precision=Full  arith_type="Signed  (2's comp)"  n_bits=10  bin_pt=0  quantization="Round  (unbiased: +/- Inf)"  overflow=Wrap  dbl_ovrd=off  block_type=mux
      settings: xl_area=[0, 0, 0, 0, 0, 0, 0]  block_version=VER_STRING_GOES_HERE
  ROM : xbsIndex_r4/ROM  depth=16  initVector=sqrt(-log( ((0:15)+0.51)'*(2.^(-1.*4)) ))  distributed_mem=Distributed memory  rst=off  init_reg=0  en=off  latency=1  arith_type=Unsigned  n_bits=9  bin_pt=7  dbl_ovrd=off  use_rpm=off  block_type=sprom
      settings: xl_area=[0, 0, 0, 0, 0, 0, 0]  block_version=VER_STRING_GOES_HERE
  ROM1 : xbsIndex_r4/ROM  depth=16  initVector=sqrt(-log( ((0:15)+0.51)'*(2.^(-2.*4)) ))  distributed_mem=Distributed memory  rst=off  init_reg=0  en=off  latency=1  arith_type=Unsigned  n_bits=9  bin_pt=7  dbl_ovrd=off  use_rpm=off  block_type=sprom
      settings: xl_area=[0, 0, 0, 0, 0, 0, 0]  block_version=VER_STRING_GOES_HERE
  ROM2 : xbsIndex_r4/ROM  depth=16  initVector=sqrt(-log( ((0:15)+0.51)'*(2.^(-3.*4)) ))  distributed_mem=Distributed memory  rst=off  init_reg=0  en=off  latency=1  arith_type=Unsigned  n_bits=9  bin_pt=7  dbl_ovrd=off  use_rpm=off  block_type=sprom
      settings: xl_area=[0, 0, 0, 0, 0, 0, 0]  block_version=VER_STRING_GOES_HERE
  ROM3 : xbsIndex_r4/ROM  depth=16  initVector=sqrt(-log( ((0:15)+0.51)'*(2.^(-4.*4)) ))  distributed_mem=Distributed memory  rst=off  init_reg=0  en=off  latency=1  arith_type=Unsigned  n_bits=9  bin_pt=7  dbl_ovrd=off  use_rpm=off  block_type=sprom
      settings: xl_area=[0, 0, 0, 0, 0, 0, 0]  block_version=VER_STRING_GOES_HERE
  ROM4 : xbsIndex_r4/ROM  depth=16  initVector=sqrt(-log( ((0:15)+0.51)'*(2.^(-5.*4)) ))  distributed_mem=Distributed memory  rst=off  init_reg=0  en=off  latency=1  arith_type=Unsigned  n_bits=9  bin_pt=7  dbl_ovrd=off  use_rpm=off  block_type=sprom
      settings: xl_area=[0, 0, 0, 0, 0, 0, 0]  block_version=VER_STRING_GOES_HERE
  ROM6 : xbsIndex_r4/ROM  depth=16  initVector=[0 1 0 2 0 1 0 3 0 1 0 2 0 1 0 4]  distributed_mem=Block RAM  rst=off  init_reg=0  en=off  latency=2  arith_type=Unsigned  n_bits=3  bin_pt=0  dbl_ovrd=off  use_rpm=off  block_type=sprom
      settings: xl_area=[0, 0, 0, 0, 0, 0, 0]  block_version=VER_STRING_GOES_HERE
  iszero : Subsystem
  iszero1 : Subsystem
  iszero2 : Subsystem
  iszero3 : Subsystem
  lfsr_17_2 : Subsystem  mask(lfsr_17){init=init1}
      mask prompts: init "init(17:1)"
  lfsr_25_2 : Subsystem  mask(lfsr_25){init=init2}
      mask prompts: init "init(25:1)"
  lfsr_29_2 : Subsystem  mask(lfsr_29){init=init3}
      mask prompts: init "init(29:1)"
  lfsr_31_2 : Subsystem  mask(lfsr_31){init=init4}
      mask prompts: init "init(31:1)"
  lfsr_41_2 : Subsystem  mask(lfsr_41){init=init5}
      mask prompts: init "init(41:1)"
  f(s') : Outport  OutDataType=sfix(16)  OutScaling=2^0
  wires:
  iszero/1(eq) -> Concat/2
  lfsr_31_2/1(" ") -> ROM/1, iszero/1(" ")
  lfsr_41_2/1(" ") -> iszero1/1(" "), ROM1/1
  lfsr_17_2/1(" ") -> ROM2/1, iszero2/1(" ")
  lfsr_25_2/1(" ") -> ROM3/1, iszero3/1(" ")
  ROM6/1 -> Mux5/1
  Concat/1 -> Concat1/2
  Concat1/1 -> Concat2/2
  ROM/1 -> Delay/1
  ROM1/1 -> Delay1/1
  Concat2/1 -> ROM6/1
  ROM2/1 -> Delay2/1
  ROM3/1 -> Delay3/1
  ROM4/1 -> Delay4/1
  iszero1/1(eq) -> Concat/1
  iszero2/1(eq) -> Concat1/1
  iszero3/1(eq) -> Concat2/1
  Mux5/1 -> f(s')/1
  Delay4/1 -> Mux5/6
  Delay3/1 -> Mux5/5
  Delay2/1 -> Mux5/4
  Delay1/1 -> Mux5/3
  Delay/1 -> Mux5/2
  lfsr_29_2/1(" ") -> ROM4/1
  reset/1 -> lfsr_41_2/1(reset), lfsr_17_2/1(reset), lfsr_25_2/1(" reset"), lfsr_29_2/1(reset), lfsr_31_2/1(reset)

== system xrbsComm_r4/White Gaussian  Noise Generator/Box-Muller4/g2 ==
  reset : Inport  OutDataType=sfix(16)  OutScaling=2^0
  Delay : xbsIndex_r4/Delay  en=off  latency=2  dbl_ovrd=off  reg_retiming=off  block_type=delay
      settings: infoedit="Delay line having  configurable length.<P><P>Hardware notes: A delay line is a chain, each link of which is an SRL16 followed by a flip-flop. If register retiming is enabled, the delay line is a chain of flip-flops."  xl_area=[0, 0, 0, 0, 0, 0, 0]  block_version=VER_STRING_GOES_HERE
  Delay1 : xbsIndex_r4/Delay  en=off  latency=1  dbl_ovrd=off  reg_retiming=off  block_type=delay
      settings: infoedit="Delay line having  configurable length.<P><P>Hardware notes: A delay line is a chain, each link of which is an SRL16 followed by a flip-flop. If register retiming is enabled, the delay line is a chain of flip-flops."  xl_area=[0, 0, 0, 0, 0, 0, 0]  block_version=VER_STRING_GOES_HERE
  ROM : xbsIndex_r4/ROM  depth=256  initVector=sqrt(2) * cos(pi*((0:255) + 0.5)*2^(-8))  distributed_mem=Block RAM  rst=off  init_reg=0  en=off  latency=1  arith_type="Signed  (2's comp)"  n_bits=10  bin_pt=8  dbl_ovrd=off  use_rpm=off  block_type=sprom
      settings: xl_area=[0, 0, 0, 0, 0, 0, 0]  block_version=VER_STRING_GOES_HERE
  lfsr_47_5 : Subsystem  mask(lfsr_47){init=init}
      mask prompts: init "init(47:1)"
  g(s') : Outport  OutDataType=sfix(16)  OutScaling=2^0
  wires:
  Delay1/1 -> ROM/1
  ROM/1 -> Delay/1
  lfsr_47_5/1(" ") -> Delay1/1
  Delay/1 -> g(s')/1
  reset/1 -> lfsr_47_5/1(reset)

== system xrbsComm_r4/White Gaussian  Noise Generator/Box-Muller1/f/iszero ==
  " " : Inport  OutDataType=sfix(16)  OutScaling=2^0
  Constant : xbsIndex_r4/Constant  arith_type=Unsigned  const=0  n_bits=4  bin_pt=0  explicit_period=off  period=1  equ=P=C  opselect=C  inp2=PCIN>>17  opr=+  inp1=P  carry=CIN  dbl_ovrd=off  block_type=constant
      settings: block_version=VER_STRING_GOES_HERE
  sel1 : xbsIndex_r4/Relational  mode=a=b  en=off  latency=1  dbl_ovrd=off  block_type=relational
      settings: xl_area=[0, 0, 0, 0, 0, 0, 0]  block_version=VER_STRING_GOES_HERE
  eq : Outport  OutDataType=sfix(16)  OutScaling=2^0
  wires:
  Constant/1 -> sel1/2
  " "/1 -> sel1/1
  sel1/1 -> eq/1

== system xrbsComm_r4/White Gaussian  Noise Generator/Box-Muller1/f/iszero1 ==
  " " : Inport  OutDataType=sfix(16)  OutScaling=2^0
  Constant : xbsIndex_r4/Constant  arith_type=Unsigned  const=0  n_bits=4  bin_pt=0  explicit_period=off  period=1  equ=P=C  opselect=C  inp2=PCIN>>17  opr=+  inp1=P  carry=CIN  dbl_ovrd=off  block_type=constant
      settings: block_version=VER_STRING_GOES_HERE
  sel2 : xbsIndex_r4/Relational  mode=a=b  en=off  latency=1  dbl_ovrd=off  block_type=relational
      settings: xl_area=[0, 0, 0, 0, 0, 0, 0]  block_version=VER_STRING_GOES_HERE
  eq : Outport  OutDataType=sfix(16)  OutScaling=2^0
  wires:
  Constant/1 -> sel2/2
  " "/1 -> sel2/1
  sel2/1 -> eq/1

== system xrbsComm_r4/White Gaussian  Noise Generator/Box-Muller1/f/iszero2 ==
  " " : Inport  OutDataType=sfix(16)  OutScaling=2^0
  Constant : xbsIndex_r4/Constant  arith_type=Unsigned  const=0  n_bits=4  bin_pt=0  explicit_period=off  period=1  equ=P=C  opselect=C  inp2=PCIN>>17  opr=+  inp1=P  carry=CIN  dbl_ovrd=off  block_type=constant
      settings: block_version=VER_STRING_GOES_HERE
  sel3 : xbsIndex_r4/Relational  mode=a=b  en=off  latency=1  dbl_ovrd=off  block_type=relational
      settings: xl_area=[0, 0, 0, 0, 0, 0, 0]  block_version=VER_STRING_GOES_HERE
  eq : Outport  OutDataType=sfix(16)  OutScaling=2^0
  wires:
  Constant/1 -> sel3/2
  " "/1 -> sel3/1
  sel3/1 -> eq/1

== system xrbsComm_r4/White Gaussian  Noise Generator/Box-Muller1/f/iszero3 ==
  " " : Inport  OutDataType=sfix(16)  OutScaling=2^0
  Constant : xbsIndex_r4/Constant  arith_type=Unsigned  const=0  n_bits=4  bin_pt=0  explicit_period=off  period=1  equ=P=C  opselect=C  inp2=PCIN>>17  opr=+  inp1=P  carry=CIN  dbl_ovrd=off  block_type=constant
      settings: block_version=VER_STRING_GOES_HERE
  sel4 : xbsIndex_r4/Relational  mode=a=b  en=off  latency=1  dbl_ovrd=off  block_type=relational
      settings: xl_area=[0, 0, 0, 0, 0, 0, 0]  block_version=VER_STRING_GOES_HERE
  eq : Outport  OutDataType=sfix(16)  OutScaling=2^0
  wires:
  Constant/1 -> sel4/2
  " "/1 -> sel4/1
  sel4/1 -> eq/1

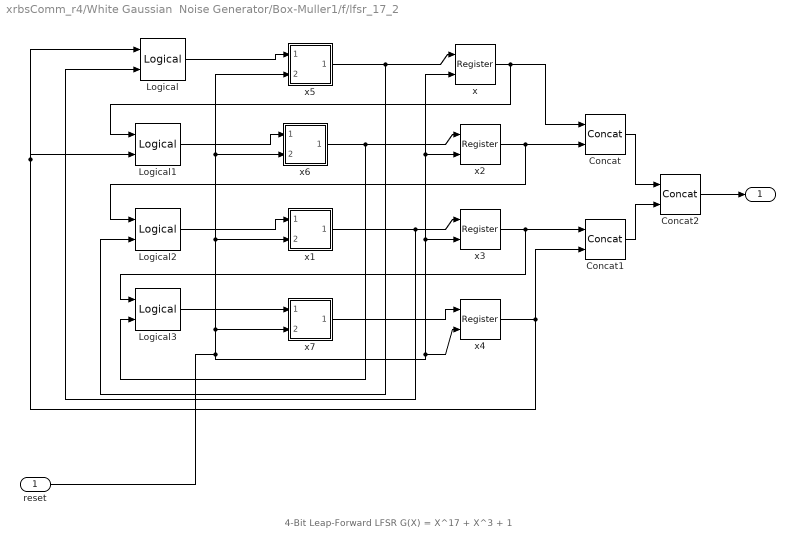
== system xrbsComm_r4/White Gaussian  Noise Generator/Box-Muller1/f/lfsr_17_2 ==
  note: 4-Bit Leap-Forward LFSR G(X) = X^17 + X^3 + 1
  reset : Inport  OutDataType=sfix(16)  OutScaling=2^0
  Concat : xbsIndex_r4/Concat  num_inputs=2  dbl_ovrd=off  block_type=concat
      settings: block_version=VER_STRING_GOES_HERE
  Concat1 : xbsIndex_r4/Concat  num_inputs=2  dbl_ovrd=off  block_type=concat
      settings: block_version=VER_STRING_GOES_HERE
  Concat2 : xbsIndex_r4/Concat  num_inputs=2  dbl_ovrd=off  block_type=concat
      settings: block_version=VER_STRING_GOES_HERE
  Logical{,1..3} (4 alike) : xbsIndex_r4/Logical  logical_function=XOR  inputs=2  en=off  latency=0  precision=User Defined  arith_type=Unsigned  n_bits=1  bin_pt=0  align_bp=on  dbl_ovrd=off  block_type=logical
      settings: xl_area=[0, 0, 0, 0, 0, 0, 0]  block_version=VER_STRING_GOES_HERE
  x : xbsIndex_r4/Register  init=init(1)  rst=on  en=off  dbl_ovrd=off  block_type=register
      settings: xl_area=[0, 0, 0, 0, 0, 0, 0]  block_version=VER_STRING_GOES_HERE
  x1 : Subsystem  mask{init=init(7:4:15)}
  x2 : xbsIndex_r4/Register  init=init(2)  rst=on  en=off  dbl_ovrd=off  block_type=register
      settings: xl_area=[0, 0, 0, 0, 0, 0, 0]  block_version=VER_STRING_GOES_HERE
  x3 : xbsIndex_r4/Register  init=init(3)  rst=on  en=off  dbl_ovrd=off  block_type=register
      settings: xl_area=[0, 0, 0, 0, 0, 0, 0]  block_version=VER_STRING_GOES_HERE
  x4 : xbsIndex_r4/Register  init=init(4)  rst=on  en=off  dbl_ovrd=off  block_type=register
      settings: xl_area=[0, 0, 0, 0, 0, 0, 0]  block_version=VER_STRING_GOES_HERE
  x5 : Subsystem  mask{init=init(5:4:17)}
  x6 : Subsystem  mask{init=init(6:4:14)}
  x7 : Subsystem  mask{init=init(8:4:16)}
  " " : Outport  OutDataType=sfix(16)  OutScaling=2^0
  wires:
  Logical/1 -> x5/1(" ")
  Logical1/1 -> x6/1(" ")
  Logical2/1 -> x1/1(" ")
  Logical3/1 -> x7/1(" ")
  x5/1(z-4) -> x/1, Logical2/2
  x6/1(z-3) -> x2/1, Logical3/2
  x1/1(z-3) -> x3/1, Logical/2
  x7/1(z-3) -> x4/1
  x/1 -> Concat/1, Logical1/1
  x2/1 -> Concat/2, Logical2/1
  Concat/1 -> Concat2/1
  x3/1 -> Concat1/1, Logical3/1
  x4/1 -> Concat1/2, Logical1/2, Logical/1
  Concat1/1 -> Concat2/2
  Concat2/1 -> " "/1
  reset/1 -> x5/2(reset), x6/2(" reset"), x1/2(" reset"), x7/2(reset), x/2, x2/2, x3/2, x4/2

== system xrbsComm_r4/White Gaussian  Noise Generator/Box-Muller1/f/lfsr_25_1 ==
  note: 4-Bit Leap-Forward LFSR G(X) = X^25 + X^3 + 1
  " reset" : Inport  OutDataType=sfix(16)  OutScaling=2^0
  Concat : xbsIndex_r4/Concat  num_inputs=2  dbl_ovrd=off  block_type=concat
      settings: block_version=VER_STRING_GOES_HERE
  Concat1 : xbsIndex_r4/Concat  num_inputs=2  dbl_ovrd=off  block_type=concat
      settings: block_version=VER_STRING_GOES_HERE
  Concat2 : xbsIndex_r4/Concat  num_inputs=2  dbl_ovrd=off  block_type=concat
      settings: block_version=VER_STRING_GOES_HERE
  Logical{,1..3} (4 alike) : xbsIndex_r4/Logical  logical_function=XOR  inputs=2  en=off  latency=0  precision=User Defined  arith_type=Unsigned  n_bits=1  bin_pt=0  align_bp=on  dbl_ovrd=off  block_type=logical
      settings: xl_area=[0, 0, 0, 0, 0, 0, 0]  block_version=VER_STRING_GOES_HERE
  x : xbsIndex_r4/Register  init=init(1)  rst=on  en=off  dbl_ovrd=off  block_type=register
      settings: xl_area=[0, 0, 0, 0, 0, 0, 0]  block_version=VER_STRING_GOES_HERE
  x1 : Subsystem  mask{init=init(7:4:23)}
  x2 : xbsIndex_r4/Register  init=init(2)  rst=on  en=off  dbl_ovrd=off  block_type=register
      settings: xl_area=[0, 0, 0, 0, 0, 0, 0]  block_version=VER_STRING_GOES_HERE
  x3 : xbsIndex_r4/Register  init=init(3)  rst=on  en=off  dbl_ovrd=off  block_type=register
      settings: xl_area=[0, 0, 0, 0, 0, 0, 0]  block_version=VER_STRING_GOES_HERE
  x4 : xbsIndex_r4/Register  init=init(4)  rst=on  en=off  dbl_ovrd=off  block_type=register
      settings: xl_area=[0, 0, 0, 0, 0, 0, 0]  block_version=VER_STRING_GOES_HERE
  x5 : Subsystem  mask{init=init(5:4:25)}
  x6 : Subsystem  mask{init=init(6:4:22)}
  x7 : Subsystem  mask{init=init(8:4:24)}
  " " : Outport  OutDataType=sfix(16)  OutScaling=2^0
  wires:
  Concat2/1 -> " "/1
  Concat1/1 -> Concat2/2
  x4/1 -> Logical/1, Logical1/2, Concat1/2
  x3/1 -> Logical3/1, Concat1/1
  Concat/1 -> Concat2/1
  x2/1 -> Logical2/1, Concat/2
  x/1 -> Concat/1, Logical1/1
  x7/1(z-5) -> x4/1
  x1/1(z-5) -> Logical/2, x3/1
  x6/1(z-5) -> Logical3/2, x2/1
  x5/1(z-6) -> Logical2/2, x/1
  Logical3/1 -> x7/1(" ")
  Logical2/1 -> x1/1(" ")
  Logical1/1 -> x6/1(" ")
  Logical/1 -> x5/1(" ")
  " reset"/1 -> x7/2(reset), x1/2(reset), x6/2(reset), x5/2(reset), x/2, x2/2, x3/2, x4/2
